simulink model "simulink_model"  (R2018b)
settings: Solver=FixedStepAuto  StartTime=0.0  StopTime=10  FixedStep=0.01  RelTol=1e-3
settings Model: OrderedModelArguments=off  Creator=leokh  LastModifiedBy=leokh

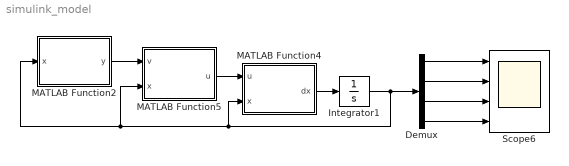
== system simulink_model ==
  Demux : Demux
  Integrator1 : Integrator  InitialCondition=[15 -15 0 0]
  MATLAB Function2 : MATLAB Function  TreatAsAtomicUnit=on
  MATLAB Function4 : MATLAB Function  TreatAsAtomicUnit=on
  MATLAB Function5 : MATLAB Function  TreatAsAtomicUnit=on
  Scope6 : Scope  NumInputPorts=4
  wires:
  MATLAB Function4/1(dx) -> Integrator1/1
  Integrator1/1 -> Demux/1, MATLAB Function4/2(x), MATLAB Function2/1(x), MATLAB Function5/2(x)
  MATLAB Function2/1(y) -> MATLAB Function5/1(v)
  Demux/1 -> Scope6/1
  MATLAB Function5/1(u) -> MATLAB Function4/1(u)
  Demux/4 -> Scope6/4
  Demux/3 -> Scope6/3
  Demux/2 -> Scope6/2

== matlab function simulink_model/MATLAB Function2 ==
  data: x input; y output
function y = hh(x)

y = x(1) + x(2);

== matlab function simulink_model/MATLAB Function4 ==
  data: u input; dx output; x input
function dx = fcn(u, x)

Ks = 1.61;
Jh = 0.0021;
m = 0.403;
g = -9.81;
h = 0.06;
Km = 0.00767;
Kg = 70;
Jl = 0.0059;
Rm = 2.6;

f = [x(3);
     x(4);
     Ks / Jh * x(2) - (Km^2 * Kg^2) / (Rm * Jh) * x(3);
     -(Ks / Jh + Ks / Jl) * x(2) + m * g * h / Jl * sin(x(1) + x(2)) + (Km^2 * Kg^2) / (Rm * Jh) * x(3)];
 
g = [0;
     0;
     (Km * Kg) / (Rm * Jh);
     -(Km * Kg) / (Rm * Jh)];

dx = f + g * u;

== matlab function simulink_model/MATLAB Function5 ==
  data: v input; x input; u output
function u = uu(v, x)

Ks = 1.61;
Jh = 0.0021;
m = 0.403;
g = -9.81;
h = 0.06;
Km = 0.00767;
Kg = 70;
Jl = 0.0059;
Rm = 2.6;

% k0 = 9999.99999999999;
% k1 = 2616.3881342812;
% k2 = 341.774343460374;
% k3 = 26.1447642353253;

k0 = 31622.7766016839;
k1 = 33624.2746746494;
k2 = 2064.83840810656;
k3 = 64.3403202992736;

u = (-Jh * Jl * Rm * (v * Jl * k0 + Jl * (x(3) + x(4)) * k1 + ...
    (-Ks * x(2) + g * h * m * sin(x(1) + x(2))) * k2 + ...
    (-Ks * x(4) + g * h * m * (x(3) + x(4)) * cos(x(1) + x(2))) * k3) + ...
    (Ks * (-((Jh + Jl) * Ks * Rm * x(2)) + Jl * Kg^2 * Km^2 * x(3)) + g * h * Jh * m * Rm * (Ks * x(2) * cos(x(1) + x(2)) + (Ks + Jl * (x(3) + x(4))^2 - g * h * m * cos(x(1) + x(2))) * sin(x(1) + x(2))))) ...
    / (Jl * Kg * Km * Ks);
